simulink model "Three_phase_bridge_rectifier_circuit_r"  (R2020a)
settings: Solver=VariableStepAuto  StartTime=0.0  StopTime=0.1  RelTol=1e-6
libraries: powerlib x9, powerlib_meascontrol x1, powerlib_extras x1
settings Model: Creator=HP  LastModifiedBy=DELL
settings DataIOCC: ReturnWorkspaceOutputs=off
settings DebuggingCC: ArithmeticOperatorsInVariantConditions=warning
settings SFSimCC: SimUseLocalCustomCode=off  CustomCodeUndefinedFunction=UseInterfaceOnly
settings RTWCC: RTWUseLocalCustomCode=off

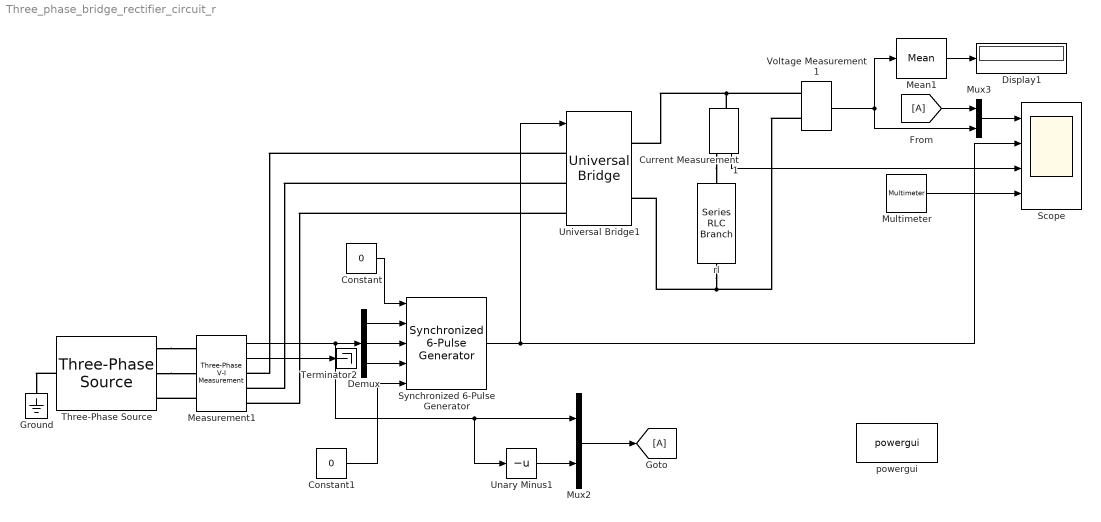
== system Three_phase_bridge_rectifier_circuit_r ==
  Constant : Constant  Value=0
  Constant1 : Constant  Value=0
  Current Measurement1 : powerlib/Measurements/Current Measurement  PhasorSimulation=off  OutputType=Complex  PSBequivalent=0
  Demux : Demux  Outputs=3
  Display1 : Display
  Ground : powerlib/Elements/Ground  LConnTagsString=a
  Mean1 : powerlib_meascontrol/Measurements/Mean  Freq=50  Vinit=0  Ts=0
  Measurement1 : powerlib/Measurements/Three-Phase V-I Measurement  VoltageMeasurement=phase-to-phase  SetLabelV=off  LabelV=Vabc  Vpu=off  VpuLL=off  CurrentMeasurement=yes  SetLabelI=off  LabelI=Iabc  Ipu=off  Pbase=100e6  Vbase=500e3  OutputType=Complex  PhasorSimulation=off  PSBequivalent=0
  Multimeter : powerlib/Measurements/Multimeter  PhasorSimulation=off  OutputType=Complex  sel=1  L=6  Gain=1  yselected={'Usw1: Universal Bridge1'};  PSBOutputType=1  PSBequivalent=0  AxesSetting=[0,0.1,-100,100]  Display=0  SavedBlockNames=-11
  Mux2 : Mux  Inputs=2
  Mux3 : Mux  Inputs=2
  Scope : Scope  NumInputPorts=4
  Synchronized 6-Pulse Generator : powerlib_extras/Control  Blocks/Synchronized 6-Pulse Generator  freq=50  pwidth=10  Double_Pulse=off
      settings: SourceProductBaseCode=PS
  Terminator2 : Terminator
  Three-Phase Source : powerlib/Electrical Sources/Three-Phase Source  InternalConnection=Yn  VoltagePhases=off  Voltage=100*sqrt(3/2)  PhaseAngle=0  Voltage_phases=[25e3 25e3 25e3]/sqrt(3)  PhaseAngles_phases=[0 -120 +120]  Frequency=50  NonIdealSource=on  SpecifyImpedance=off  Resistance=0  Inductance=0  ShortCircuitLevel=100e6  BaseVoltage=100*sqrt(3/2)  XRratio=7  BusType=swing  Pref=10e3  Qref=0  Prefabc=[10e3, 10e3, 10e3]  Qrefabc=[0, 0, 0]  Qmin=-inf  Qmax=inf
  Unary Minus1 : UnaryMinus
  Universal Bridge1 : powerlib/Power Electronics/Universal Bridge  Arms=3  SnubberResistance=1e5  SnubberCapacitance=inf  Device=Thyristors  Ron=1e-3  Lon=0  ForwardVoltages="[  0  0  ]"  ForwardVoltage=0  GTOparameters=[ 10e-6 , 20e-6 ]  IGBTparameters=[ 1e-6 , 2e-6 ]  Measurements=Device voltages  Measurements_2=None  converterType=Rectifier
  Voltage Measurement1 : powerlib/Measurements/Voltage Measurement  PhasorSimulation=off  OutputType=Complex  PSBequivalent=0
  powergui : powerlib/powergui  Priority=1  SimulationMode=Continuous  SampleTime=50e-6  frequency=60  Iterations=50  frequencyindice=50  Pbase=100e6  ErrMax=1e-4  UnitsV=kV  UnitsW=MW  buscounter=0  FunctionMessages=off  echomessages=off  EnableUseOfTLC=off  CurrentSourceSwitches=off  DisableSnubberDevices=off  DisableRonSwitches=off  DisableVfSwitches=off  DisplayEquations=off  AutomaticDiscreteSolvers=off  SolverType=Tustin/Backward Euler (TBE)  Interpol=off  ExternalGateDelay=off  methode=off  Ts=100  x0status=blocks  SPID=on  SwTol=0  HookPort=off  NonlinearTolerance=1e-4  nMaxIteration=100  ContinueOnMaxIteration=off  RestoreLinks=warning  ResistiveCurrentMeasurement=off  Frange=[0:2:500]  Ylog=off  Xlog=on  ShowGrid=off  save=off  variable=ZData  structure=0  ZoomFFT=off  StartTime=0.0  cycles=1  DisplayStyle=1  fundamental=60  FreqAxis=off  MaxFrequency=1000  frequencyindicesteady=1  RmsSteady=1  display=off
  rl : powerlib/Elements/Series RLC Branch  LConnTagsString=__new0  RConnTagsString=__new0  BranchType=R  Resistance=50  Inductance=30e-3  SetiL0=off  InitialCurrent=0  Capacitance=1e-6  Setx0=off  InitialVoltage=0  Measurements=None
  wires:
  Synchronized 6-Pulse Generator/1 -> Scope/2, Universal Bridge1/1
  Voltage Measurement1/1 -> Mean1/1, Mux3/2
  Mean1/1 -> Display1/1
  Mux2/1 -> [A]
  Constant1/1 -> Synchronized 6-Pulse Generator/5
  Constant/1 -> Synchronized 6-Pulse Generator/1
  Demux/1 -> Synchronized 6-Pulse Generator/2
  Demux/2 -> Synchronized 6-Pulse Generator/3
  Demux/3 -> Synchronized 6-Pulse Generator/4
  Measurement1/2 -> Terminator2/1
  Unary Minus1/1 -> Mux2/2
  Measurement1/1 -> Unary Minus1/1, Mux2/1, Demux/1
  Mux3/1 -> Scope/1
  Multimeter/1 -> Scope/4
  [A] -> Mux3/1
  Current Measurement1/1 -> Scope/3
  connections:
  Measurement1/LConn3 -- Three-Phase Source/RConn3
  Voltage Measurement1/LConn1 -- Current Measurement1/LConn1 -- Universal Bridge1/RConn1
  Three-Phase Source/RConn2 -- Measurement1/LConn2
  Three-Phase Source/RConn1 -- Measurement1/LConn1
  Universal Bridge1/RConn2 -- rl/LConn1 -- Voltage Measurement1/LConn2
  Current Measurement1/RConn1 -- rl/RConn1
  Universal Bridge1/LConn1 -- Measurement1/RConn1
  Universal Bridge1/LConn2 -- Measurement1/RConn2
  Universal Bridge1/LConn3 -- Measurement1/RConn3
  Three-Phase Source/LConn1 -- Ground/LConn1
